simulink model "sf_tlbefore"  (R2017b)
settings: Solver=ode45  StartTime=0.0  StopTime=20  MaxStep=.01  RelTol=1e-3  EnableMultiTasking=on
settings Model: FPTRunName=Active  ExtModeAutoUpdateStatusClock=off  Creator=The MathWorks, Inc.  LastModifiedBy=The MathWorks, Inc.
settings DataIOCC: LimitDataPoints=on  SaveFormat=Array
settings OptimizationCC: BooleanDataType=off  ExpressionDepthLimit=2147483647  InitFltsAndDblsToZero=on  EfficientMapNaN2IntZero=off  LifeSpan=inf
settings DebuggingCC: SaveWithParameterizedLinksMsg=none  UnderspecifiedInitializationDetection=Classic  MergeDetectMultiDrivingBlocksExec=none  SignalResolutionControl=TryResolveAllWithWarning  MultiTaskDSMMsg=warning  MultiTaskCondExecSysMsg=none  FcnCallInpInsideContextMsg=warning  StateNameClashWarn=warning  StrictBusMsg=None  SFUnexpectedBacktrackingDiag=warning  SFNoUnconditionalDefaultTransitionDiag=warning  SFExecutionAtInitializationDiag=none
settings HardwareCC: ProdBitPerPointer=32  ProdBitPerSizeT=32  ProdBitPerPtrDiffT=32  ProdLargestAtomicFloat=None  ProdIntDivRoundTo=Undefined  ProdEndianess=Unspecified  ProdWordSize=32  ProdHWDeviceType=32-bit Generic  TargetUnknown=on
settings ModelReferenceCC: PropagateSignalLabelsOutOfModel=off
settings SFSimCC: SimParseCustomCode=off
settings CodeAppCC: StateflowObjectComments=on
settings GRTTargetCC: TargetFcnLib=ansi_tfl_tmw.mat  TargetLangStandard=C89/C90 (ANSI)  GeneratePreprocessorConditionals=Disable all  CombineOutputUpdateFcns=off  GRTInterface=on
settings ConfigComp: CovMetricSettings=dcmtr  CovHtmlReporting=on  CovSaveCumulativeToWorkspaceVar=on  CovSaveSingleToWorkspaceVar=on  CovExternalEMLEnable=off  CovSFcnEnable=off

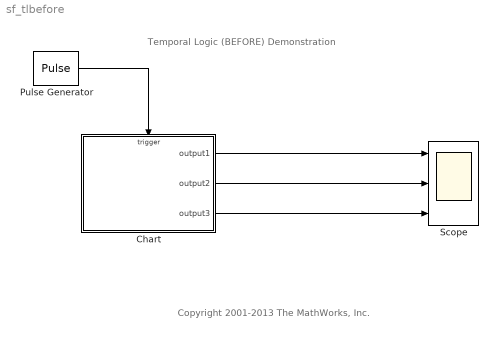
== system sf_tlbefore ==
  note: Temporal Logic (BEFORE) Demonstration
  note: Copyright 2001-2013 The MathWorks, Inc.
  Chart : Stateflow chart  TreatAsAtomicUnit=on
  Pulse Generator : DiscretePulseGenerator  PulseType=Time based  Period=1  PulseWidth=50
  Scope : Scope  NumInputPorts=3
  wires:
  Pulse Generator/1 -> Chart/Trigger
  Chart/1(output1) -> Scope/1
  Chart/2(output2) -> Scope/2
  Chart/3(output3) -> Scope/3

== stateflow chart sf_tlbefore/Chart ==
  state One [parallel]
    settings: executionOrder=1
    state A_state
      on count:signal_one = signal_one + 1;
    A_state -> (junction 14) : before(10,count)[signal_one<5]{output1=1;}
    (junction 14) -> A_state
  state Two [parallel]
    settings: executionOrder=2
    state B_state
      on count:signal_two = signal_two + 1;
    B_state -> (junction 15) : before(20,count)[signal_two>10]{output2=1;}
    (junction 15) -> B_state
  state Three [parallel]
    settings: executionOrder=3
    state C_state
      on count:signal_three = signal_three + 1;
    C_state -> (junction 16) : before(10,count)[signal_three>11]{output3=1;}
    (junction 16) -> C_state
  (default) -> A_state : {signal_one=0;signal_two=0;signal_three=0;}
  data: output1 output double; signal_three local double; output2 output double; output3 output double; signal_one local double; signal_two local double
  events: count input RISING_EDGE_EVENT
